simulink model "CTC_3PPP"  (R2018b)
settings: Solver=ode3  StartTime=0.0  StopTime=7  FixedStep=1e-3  RelTol=1e-3  EnableMultiTasking=on
undefined symbols (not defined in the file or in its folder): X, Y, Z
libraries: sm_lib x53, nesl_utility x13, simulink x2
(part 2 of 2)

== system CTC_3PPP/Mechanical/Mechanical/L2_6_RIGID ==
  ReferenceFrame : sm_lib/Frames and Transforms/Reference Frame
  Solid : sm_lib/Body Elements/Solid  InertiaType=Custom  Mass=7.3903600000000003  MassUnits=kg  CenterOfMass=[-300 -10 0]  CenterOfMassUnits=mm  MomentsOfInertia=[4161.6100000000006 267638 263969]  MomentsOfInertiaUnits=kg*mm^2  ProductsOfInertia=[0 0 0]  ProductsOfInertiaUnits=kg*mm^2  BasedOnType=Density  Density=1000  DensityUnits=kg/(m^3)  DoExposeReferenceFrame=on  SerializedFrames=<Frames/>  GraphicType=FromGeometry  MarkerShape=Sphere  MarkerSize=10  MarkerSizeUnits=m  GraphicVisPropType=SimpleVisualProperties  GraphicDiffuseColor=[0.909804 0.443137 0.0313725]  GraphicSpecularColor=[0.5 0.5 0.5 1.0]  GraphicAmbientColor=[0.15 0.15 0.15 1.0]  GraphicEmissiveColor=[0.0 0.0 0.0 1.0]  GraphicShininess=75  GraphicOpacity=1  GeometryShape=FromFile  RectangleSize=[1 1]  RectangleSizeUnits=m  BrickDimensions=[1 1 1]  BrickDimensionUnits=m  CylinderRadius=1  CylinderRadiusUnits=m  CylinderLength=1  CylinderLengthUnits=m  SphereRadius=1  SphereRadiusUnits=m  EllipsoidRadii=[1 1 1]  EllipsoidRadiiUnits=m  ExtrusionCrossSection=[1 1; -1 1; -1 -1; 1 -1]  ExtrusionCrossSectionUnits=m  ExtrusionLength=1  ExtrusionLengthUnits=m  PolygonNumSides=3  PolygonOuterRadius=1  PolygonOuterRadiusUnits=m  ExtGeomFileType=STL  ExtGeomFileName=L2_Default_sldprt.STL  ExtGeomFileUnits=mm  RevolutionCrossSection=[1 1; 1 -1; 2 -1; 2 1]  RevolutionCrossSectionUnits=m  RevolutionExtent=Full  RevolutionAngle=180  RevolutionAngleUnits=deg
  Transform : sm_lib/Frames and Transforms/Rigid Transform  TranslationMethod=Cartesian  TranslationStandardOffset=0  TranslationLengthUnit=mm  TranslationStandardAxis=+Z  TranslationCartesianOffset=[-600.00300519535062 20.000000000004142 -0.0012441245004310986]  TranslationROffset=0  TranslationROffsetUnits=m  TranslationZOffset=0  TranslationZOffsetUnits=m  TranslationThetaOffset=0  TranslationThetaOffsetUnits=deg  RotationMethod=ArbitraryAxis  RotationAngleUnits=rad  RotationStandardAxis=+Z  RotationAngle=2.0943951023931953  RotationArbitraryAxis=[0.57735026918962584 -0.57735026918962595 0.57735026918962573]  FollAlignAxisA=+X  BaseAlignAxisA=+Y  FollAlignAxisB=+Y  BaseAlignAxisB=+Z  RotationSequenceAxes=FollowerAxes  RotationSequence=XYX  RotationSequenceAngles=[0 0 0]  RotationSequenceAnglesUnits=deg  RotationMatrix=[1 0 0; 0 1 0; 0 0 1]
  Transform1 : sm_lib/Frames and Transforms/Rigid Transform  TranslationMethod=Cartesian  TranslationStandardOffset=0  TranslationLengthUnit=mm  TranslationStandardAxis=+Z  TranslationCartesianOffset=[0 0 0]  TranslationROffset=0  TranslationROffsetUnits=m  TranslationZOffset=0  TranslationZOffsetUnits=m  TranslationThetaOffset=0  TranslationThetaOffsetUnits=deg  RotationMethod=ArbitraryAxis  RotationAngleUnits=rad  RotationStandardAxis=+Z  RotationAngle=2.0943951023931953  RotationArbitraryAxis=[0.57735026918962584 -0.57735026918962584 0.57735026918962584]  FollAlignAxisA=+X  BaseAlignAxisA=+Y  FollAlignAxisB=+Y  BaseAlignAxisB=+Z  RotationSequenceAxes=FollowerAxes  RotationSequence=XYX  RotationSequenceAngles=[0 0 0]  RotationSequenceAnglesUnits=deg  RotationMatrix=[1 0 0; 0 1 0; 0 0 1]
  F : PMIOPort  Side=Left
  F1 : PMIOPort  Port=2  Side=Right
  connections:
  Solid/RConn1 -- ReferenceFrame/RConn1 -- Transform/LConn1 -- Transform1/LConn1
  Transform/RConn1 -- F/RConn1
  Transform1/RConn1 -- F1/RConn1

== system CTC_3PPP/Mechanical/Mechanical/de2_5_RIGID ==
  ReferenceFrame : sm_lib/Frames and Transforms/Reference Frame
  Solid : sm_lib/Body Elements/Solid  InertiaType=Custom  Mass=5.2339599999999997  MassUnits=kg  CenterOfMass=[0 145.71899999999999 1.0172299999999999e-12]  CenterOfMassUnits=mm  MomentsOfInertia=[33998.800000000003 21791.899999999998 33998.800000000003]  MomentsOfInertiaUnits=kg*mm^2  ProductsOfInertia=[0 0 0]  ProductsOfInertiaUnits=kg*mm^2  BasedOnType=Density  Density=1000  DensityUnits=kg/(m^3)  DoExposeReferenceFrame=on  SerializedFrames=<Frames/>  GraphicType=FromGeometry  MarkerShape=Sphere  MarkerSize=10  MarkerSizeUnits=m  GraphicVisPropType=SimpleVisualProperties  GraphicDiffuseColor=[0.792157 0.819608 0.933333]  GraphicSpecularColor=[0.5 0.5 0.5 1.0]  GraphicAmbientColor=[0.15 0.15 0.15 1.0]  GraphicEmissiveColor=[0.0 0.0 0.0 1.0]  GraphicShininess=75  GraphicOpacity=1  GeometryShape=FromFile  RectangleSize=[1 1]  RectangleSizeUnits=m  BrickDimensions=[1 1 1]  BrickDimensionUnits=m  CylinderRadius=1  CylinderRadiusUnits=m  CylinderLength=1  CylinderLengthUnits=m  SphereRadius=1  SphereRadiusUnits=m  EllipsoidRadii=[1 1 1]  EllipsoidRadiiUnits=m  ExtrusionCrossSection=[1 1; -1 1; -1 -1; 1 -1]  ExtrusionCrossSectionUnits=m  ExtrusionLength=1  ExtrusionLengthUnits=m  PolygonNumSides=3  PolygonOuterRadius=1  PolygonOuterRadiusUnits=m  ExtGeomFileType=STL  ExtGeomFileName=de2_Default_sldprt.STL  ExtGeomFileUnits=mm  RevolutionCrossSection=[1 1; 1 -1; 2 -1; 2 1]  RevolutionCrossSectionUnits=m  RevolutionExtent=Full  RevolutionAngle=180  RevolutionAngleUnits=deg
  Transform : sm_lib/Frames and Transforms/Rigid Transform  TranslationMethod=Cartesian  TranslationStandardOffset=0  TranslationLengthUnit=mm  TranslationStandardAxis=+Z  TranslationCartesianOffset=[0 0 0]  TranslationROffset=0  TranslationROffsetUnits=m  TranslationZOffset=0  TranslationZOffsetUnits=m  TranslationThetaOffset=0  TranslationThetaOffsetUnits=deg  RotationMethod=ArbitraryAxis  RotationAngleUnits=rad  RotationStandardAxis=+Z  RotationAngle=2.0943951023931913  RotationArbitraryAxis=[-0.57735026918962451 -0.57735026918962451 -0.57735026918962828]  FollAlignAxisA=+X  BaseAlignAxisA=+Y  FollAlignAxisB=+Y  BaseAlignAxisB=+Z  RotationSequenceAxes=FollowerAxes  RotationSequence=XYX  RotationSequenceAngles=[0 0 0]  RotationSequenceAnglesUnits=deg  RotationMatrix=[1 0 0; 0 1 0; 0 0 1]
  F1 : PMIOPort  Side=Left
  F : PMIOPort  Port=2  Side=Right
  connections:
  Solid/RConn1 -- ReferenceFrame/RConn1 -- Transform/LConn1 -- F1/RConn1
  Transform/RConn1 -- F/RConn1

== system CTC_3PPP/Mechanical/Mechanical/de2_6_RIGID ==
  ReferenceFrame : sm_lib/Frames and Transforms/Reference Frame
  Solid : sm_lib/Body Elements/Solid  InertiaType=Custom  Mass=5.2339599999999997  MassUnits=kg  CenterOfMass=[0 145.71899999999999 1.0172299999999999e-12]  CenterOfMassUnits=mm  MomentsOfInertia=[33998.800000000003 21791.899999999998 33998.800000000003]  MomentsOfInertiaUnits=kg*mm^2  ProductsOfInertia=[0 0 0]  ProductsOfInertiaUnits=kg*mm^2  BasedOnType=Density  Density=1000  DensityUnits=kg/(m^3)  DoExposeReferenceFrame=on  SerializedFrames=<Frames/>  GraphicType=FromGeometry  MarkerShape=Sphere  MarkerSize=10  MarkerSizeUnits=m  GraphicVisPropType=SimpleVisualProperties  GraphicDiffuseColor=[0.792157 0.819608 0.933333]  GraphicSpecularColor=[0.5 0.5 0.5 1.0]  GraphicAmbientColor=[0.15 0.15 0.15 1.0]  GraphicEmissiveColor=[0.0 0.0 0.0 1.0]  GraphicShininess=75  GraphicOpacity=1  GeometryShape=FromFile  RectangleSize=[1 1]  RectangleSizeUnits=m  BrickDimensions=[1 1 1]  BrickDimensionUnits=m  CylinderRadius=1  CylinderRadiusUnits=m  CylinderLength=1  CylinderLengthUnits=m  SphereRadius=1  SphereRadiusUnits=m  EllipsoidRadii=[1 1 1]  EllipsoidRadiiUnits=m  ExtrusionCrossSection=[1 1; -1 1; -1 -1; 1 -1]  ExtrusionCrossSectionUnits=m  ExtrusionLength=1  ExtrusionLengthUnits=m  PolygonNumSides=3  PolygonOuterRadius=1  PolygonOuterRadiusUnits=m  ExtGeomFileType=STL  ExtGeomFileName=de2_Default_sldprt.STL  ExtGeomFileUnits=mm  RevolutionCrossSection=[1 1; 1 -1; 2 -1; 2 1]  RevolutionCrossSectionUnits=m  RevolutionExtent=Full  RevolutionAngle=180  RevolutionAngleUnits=deg
  Transform : sm_lib/Frames and Transforms/Rigid Transform  TranslationMethod=Cartesian  TranslationStandardOffset=0  TranslationLengthUnit=mm  TranslationStandardAxis=+Z  TranslationCartesianOffset=[0 0 0]  TranslationROffset=0  TranslationROffsetUnits=m  TranslationZOffset=0  TranslationZOffsetUnits=m  TranslationThetaOffset=0  TranslationThetaOffsetUnits=deg  RotationMethod=ArbitraryAxis  RotationAngleUnits=rad  RotationStandardAxis=+Z  RotationAngle=2.0943951023931913  RotationArbitraryAxis=[-0.57735026918962451 -0.57735026918962451 -0.57735026918962828]  FollAlignAxisA=+X  BaseAlignAxisA=+Y  FollAlignAxisB=+Y  BaseAlignAxisB=+Z  RotationSequenceAxes=FollowerAxes  RotationSequence=XYX  RotationSequenceAngles=[0 0 0]  RotationSequenceAnglesUnits=deg  RotationMatrix=[1 0 0; 0 1 0; 0 0 1]
  F1 : PMIOPort  Side=Left
  F : PMIOPort  Port=2  Side=Right
  connections:
  Solid/RConn1 -- ReferenceFrame/RConn1 -- Transform/LConn1 -- F1/RConn1
  Transform/RConn1 -- F/RConn1

== system CTC_3PPP/Mechanical/Mechanical/de2_7_RIGID ==
  ReferenceFrame : sm_lib/Frames and Transforms/Reference Frame
  Solid : sm_lib/Body Elements/Solid  InertiaType=Custom  Mass=5.2339599999999997  MassUnits=kg  CenterOfMass=[0 145.71899999999999 1.0172299999999999e-12]  CenterOfMassUnits=mm  MomentsOfInertia=[33998.800000000003 21791.899999999998 33998.800000000003]  MomentsOfInertiaUnits=kg*mm^2  ProductsOfInertia=[0 0 0]  ProductsOfInertiaUnits=kg*mm^2  BasedOnType=Density  Density=1000  DensityUnits=kg/(m^3)  DoExposeReferenceFrame=on  SerializedFrames=<Frames/>  GraphicType=FromGeometry  MarkerShape=Sphere  MarkerSize=10  MarkerSizeUnits=m  GraphicVisPropType=SimpleVisualProperties  GraphicDiffuseColor=[0.792157 0.819608 0.933333]  GraphicSpecularColor=[0.5 0.5 0.5 1.0]  GraphicAmbientColor=[0.15 0.15 0.15 1.0]  GraphicEmissiveColor=[0.0 0.0 0.0 1.0]  GraphicShininess=75  GraphicOpacity=1  GeometryShape=FromFile  RectangleSize=[1 1]  RectangleSizeUnits=m  BrickDimensions=[1 1 1]  BrickDimensionUnits=m  CylinderRadius=1  CylinderRadiusUnits=m  CylinderLength=1  CylinderLengthUnits=m  SphereRadius=1  SphereRadiusUnits=m  EllipsoidRadii=[1 1 1]  EllipsoidRadiiUnits=m  ExtrusionCrossSection=[1 1; -1 1; -1 -1; 1 -1]  ExtrusionCrossSectionUnits=m  ExtrusionLength=1  ExtrusionLengthUnits=m  PolygonNumSides=3  PolygonOuterRadius=1  PolygonOuterRadiusUnits=m  ExtGeomFileType=STL  ExtGeomFileName=de2_Default_sldprt.STL  ExtGeomFileUnits=mm  RevolutionCrossSection=[1 1; 1 -1; 2 -1; 2 1]  RevolutionCrossSectionUnits=m  RevolutionExtent=Full  RevolutionAngle=180  RevolutionAngleUnits=deg
  Transform : sm_lib/Frames and Transforms/Rigid Transform  TranslationMethod=Cartesian  TranslationStandardOffset=0  TranslationLengthUnit=mm  TranslationStandardAxis=+Z  TranslationCartesianOffset=[0 0 0]  TranslationROffset=0  TranslationROffsetUnits=m  TranslationZOffset=0  TranslationZOffsetUnits=m  TranslationThetaOffset=0  TranslationThetaOffsetUnits=deg  RotationMethod=ArbitraryAxis  RotationAngleUnits=rad  RotationStandardAxis=+Z  RotationAngle=2.0943951023931913  RotationArbitraryAxis=[-0.57735026918962451 -0.57735026918962451 -0.57735026918962828]  FollAlignAxisA=+X  BaseAlignAxisA=+Y  FollAlignAxisB=+Y  BaseAlignAxisB=+Z  RotationSequenceAxes=FollowerAxes  RotationSequence=XYX  RotationSequenceAngles=[0 0 0]  RotationSequenceAnglesUnits=deg  RotationMatrix=[1 0 0; 0 1 0; 0 0 1]
  F1 : PMIOPort  Side=Left
  F : PMIOPort  Port=2  Side=Right
  connections:
  Solid/RConn1 -- ReferenceFrame/RConn1 -- Transform/LConn1 -- F1/RConn1
  Transform/RConn1 -- F/RConn1

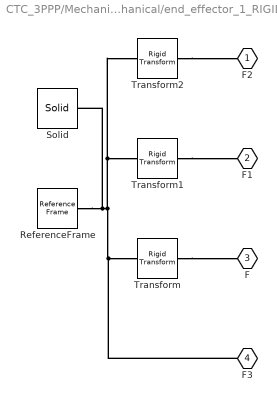
== system CTC_3PPP/Mechanical/Mechanical/end_effector_1_RIGID ==
  ReferenceFrame : sm_lib/Frames and Transforms/Reference Frame
  Solid : sm_lib/Body Elements/Solid  InertiaType=Custom  Mass=3.8378800000000002  MassUnits=kg  CenterOfMass=[0 -7.5 -1.46335e-12]  CenterOfMassUnits=mm  MomentsOfInertia=[32683.700000000004 65223.500000000007 32683.700000000004]  MomentsOfInertiaUnits=kg*mm^2  ProductsOfInertia=[0 0 0]  ProductsOfInertiaUnits=kg*mm^2  BasedOnType=Density  Density=1000  DensityUnits=kg/(m^3)  DoExposeReferenceFrame=on  SerializedFrames=<Frames/>  GraphicType=FromGeometry  MarkerShape=Sphere  MarkerSize=10  MarkerSizeUnits=m  GraphicVisPropType=SimpleVisualProperties  GraphicDiffuseColor=[0.894118 0.913725 0.929412]  GraphicSpecularColor=[0.5 0.5 0.5 1.0]  GraphicAmbientColor=[0.15 0.15 0.15 1.0]  GraphicEmissiveColor=[0.0 0.0 0.0 1.0]  GraphicShininess=75  GraphicOpacity=1  GeometryShape=FromFile  RectangleSize=[1 1]  RectangleSizeUnits=m  BrickDimensions=[1 1 1]  BrickDimensionUnits=m  CylinderRadius=1  CylinderRadiusUnits=m  CylinderLength=1  CylinderLengthUnits=m  SphereRadius=1  SphereRadiusUnits=m  EllipsoidRadii=[1 1 1]  EllipsoidRadiiUnits=m  ExtrusionCrossSection=[1 1; -1 1; -1 -1; 1 -1]  ExtrusionCrossSectionUnits=m  ExtrusionLength=1  ExtrusionLengthUnits=m  PolygonNumSides=3  PolygonOuterRadius=1  PolygonOuterRadiusUnits=m  ExtGeomFileType=STL  ExtGeomFileName=end-effector_Default_sldprt.STL  ExtGeomFileUnits=mm  RevolutionCrossSection=[1 1; 1 -1; 2 -1; 2 1]  RevolutionCrossSectionUnits=m  RevolutionExtent=Full  RevolutionAngle=180  RevolutionAngleUnits=deg
  Transform : sm_lib/Frames and Transforms/Rigid Transform  TranslationMethod=Cartesian  TranslationStandardOffset=0  TranslationLengthUnit=mm  TranslationStandardAxis=+Z  TranslationCartesianOffset=[-173.2045872608081 -15.00000000000081 -99.999473127677447]  TranslationROffset=0  TranslationROffsetUnits=m  TranslationZOffset=0  TranslationZOffsetUnits=m  TranslationThetaOffset=0  TranslationThetaOffsetUnits=deg  RotationMethod=ArbitraryAxis  RotationAngleUnits=rad  RotationStandardAxis=+Z  RotationAngle=2.0943951023931953  RotationArbitraryAxis=[0.57735026918962584 -0.57735026918962584 0.57735026918962584]  FollAlignAxisA=+X  BaseAlignAxisA=+Y  FollAlignAxisB=+Y  BaseAlignAxisB=+Z  RotationSequenceAxes=FollowerAxes  RotationSequence=XYX  RotationSequenceAngles=[0 0 0]  RotationSequenceAnglesUnits=deg  RotationMatrix=[1 0 0; 0 1 0; 0 0 1]
  Transform1 : sm_lib/Frames and Transforms/Rigid Transform  TranslationMethod=Cartesian  TranslationStandardOffset=0  TranslationLengthUnit=mm  TranslationStandardAxis=+Z  TranslationCartesianOffset=[173.20555958822573 -15.000000000000609 -99.999297526180612]  TranslationROffset=0  TranslationROffsetUnits=m  TranslationZOffset=0  TranslationZOffsetUnits=m  TranslationThetaOffset=0  TranslationThetaOffsetUnits=deg  RotationMethod=ArbitraryAxis  RotationAngleUnits=rad  RotationStandardAxis=+Z  RotationAngle=2.0943951023931957  RotationArbitraryAxis=[0.57735026918962573 -0.57735026918962573 0.57735026918962584]  FollAlignAxisA=+X  BaseAlignAxisA=+Y  FollAlignAxisB=+Y  BaseAlignAxisB=+Z  RotationSequenceAxes=FollowerAxes  RotationSequence=XYX  RotationSequenceAngles=[0 0 0]  RotationSequenceAnglesUnits=deg  RotationMatrix=[1 0 0; 0 1 0; 0 0 1]
  Transform2 : sm_lib/Frames and Transforms/Rigid Transform  TranslationMethod=Cartesian  TranslationStandardOffset=0  TranslationLengthUnit=mm  TranslationStandardAxis=+Z  TranslationCartesianOffset=[0.00019460048216402015 -14.999999999998581 200.00067808125598]  TranslationROffset=0  TranslationROffsetUnits=m  TranslationZOffset=0  TranslationZOffsetUnits=m  TranslationThetaOffset=0  TranslationThetaOffsetUnits=deg  RotationMethod=ArbitraryAxis  RotationAngleUnits=rad  RotationStandardAxis=+Z  RotationAngle=2.0943951023931953  RotationArbitraryAxis=[0.57735026918962584 -0.57735026918962584 0.57735026918962584]  FollAlignAxisA=+X  BaseAlignAxisA=+Y  FollAlignAxisB=+Y  BaseAlignAxisB=+Z  RotationSequenceAxes=FollowerAxes  RotationSequence=XYX  RotationSequenceAngles=[0 0 0]  RotationSequenceAnglesUnits=deg  RotationMatrix=[1 0 0; 0 1 0; 0 0 1]
  F2 : PMIOPort  Side=Left
  F1 : PMIOPort  Port=2  Side=Left
  F : PMIOPort  Port=3  Side=Left
  F3 : PMIOPort  Port=4  Side=Right
  connections:
  Solid/RConn1 -- ReferenceFrame/RConn1 -- Transform1/LConn1 -- Transform2/LConn1 -- F3/RConn1 -- Transform/LConn1
  Transform/RConn1 -- F/RConn1
  Transform1/RConn1 -- F1/RConn1
  Transform2/RConn1 -- F2/RConn1

== matlab function CTC_3PPP/MATLAB Function1 ==
  data: x output; teta1 input; y output; teta2 input; teta3 input; goc output; phi1 output; phi2 output; phi3 output
function  [x,y,goc,phi1,phi2,phi3]=forward1(teta1,teta2,teta3)
%% Thong so
l1=0.4;
l2=0.6;
l3=0.2;
%%
phii=[pi/6 5*pi/6 3*pi/2];
xoi=[0 1 0.5];
yoi=[0 0 sqrt(3)/2];

gama1=7*pi/6;
gama2=11*pi/6;
gama3=pi/2;
gama=[gama1; gama2; gama3;];
%%
z2=[0;0;0;];

%% giai phuong trinh tai day
coder.extrinsic('giaihe') %% chuyen C++ => matlab function
z2=giaihe(teta1,teta2,teta3);
x=z2(1);
y=z2(2);
goc=z2(3);
tam=[0; 0; 0;];
%% Tinh phi
phi=[0; 0; 0;];
xci=[0; 0; 0;];
yci=[0; 0; 0;];
for i=1:3
    xci(i)=x+l3*cos(goc+gama(i))-xoi(i);
    yci(i)=y+l3*sin(goc+gama(i))-yoi(i);
    tam(i)=(l1^2+l2^2-xci(i)^2-yci(i)^2)/(2*l1*l2);
    phi(i)=acos(tam(i))-pi;
end
%%
xc1=xci(1);
xc2=xci(2);
xc3=xci(3);
yc1=yci(1);
yc2=yci(2);
yc3=yci(3);
phi1=phi(1);
phi2=phi(2);
phi3=phi(3);

== matlab function CTC_3PPP/Mechanical/Mechanical/Coulomb & Viscous Friction3/Embedded MATLAB Function ==
  data: u input; y output
function y = Sat(u)

if (abs(u)>0.01)
    y = sign(u);
else
    y = u/0.01;
end

== matlab function CTC_3PPP/Mechanical/Mechanical/Coulomb & Viscous Friction1/Embedded MATLAB Function ==
  data: u input; y output
function y = Sat(u)

if (abs(u)>0.01)
    y = sign(u);
else
    y = u/0.01;
end

== matlab function CTC_3PPP/Mechanical/Mechanical/Coulomb & Viscous Friction2/Embedded MATLAB Function ==
  data: u input; y output
function y = Sat(u)

if (abs(u)>0.01)
    y = sign(u);
else
    y = u/0.01;
end

== matlab function CTC_3PPP/MATLAB Function2 ==
  settings: updateMethod=DISCRETE
  data: xp input; To1 output; yp input; anpha input; teta1 input; teta2 input; teta3 input; phi1 input; phi2 input; phi3 input; teta1_dot input; teta2_dot input; teta3_dot input; teta1d input; teta2d input; teta3d input; teta1d_dot input; teta2d_dot input; teta3d_dot input; teta1d_2dot input; teta2d_2dot input; teta3d_2dot input; To2 output; To3 output
function [To1,To2,To3] = Dynamic(xp,yp,anpha,teta1,teta2,teta3,phi1,phi2,phi3,teta1_dot,teta2_dot,teta3_dot,teta1d,teta2d,teta3d,teta1d_dot,teta2d_dot,teta3d_dot,teta1d_2dot,teta2d_2dot,teta3d_2dot)


%% Thong so
l1=0.4;
l2=0.6;
l3=0.2;
%%
gama1=pi/6+anpha;
gama2=5*pi/6+anpha;
gama3=3*pi/2+anpha;
gama=[gama1; gama2; gama3;];

%%
m1=5.11836;I1=91391*10^-6;% kg/m^2;
m2=7.39036;I2=267638*10^-6; % kg/m^2;
mp=3.83788; Ip=65223*10^-6% % kg/m^2; - end-effector

%%
xoi=[0 1 0.5];
yoi=[0 0 sqrt(3)/2];
%%
tetaout1=teta1;
tetaout2=teta2;
tetaout3=teta3;
%%
teta=[teta1; teta2; teta3;];
phi=[phi1; phi2; phi3;];
z=[xp; yp; anpha;];
z_dot=[0; 0; 0;];
z_2dot=[0; 0; 0;];
%%
teta_dot=[teta1_dot; teta2_dot; teta3_dot;];
teta_2dot=[0; 0; 0;];
%% Tinh Jz1*z_dot=Jo*teta_dot;
%% z_dot= inv(Jz1)*Jo*teta_dot
az1=[0 0 0];
bz1=[0 0 0];
cz1=[0 0 0];
dz1=[0 0 0];

for i=1:3
    az1(i)=cos(teta(i)+phi(i));
    bz1(i)=sin(teta(i)+phi(i));
    cz1(i)=-l3*sin(teta(i)+phi(i)-gama(i));
    dz1(i)=l1*sin(phi(i));
end
Jz1=[az1(1) bz1(1) cz1(1);
     az1(2) bz1(2) cz1(2);
     az1(3) bz1(3) cz1(3);];
 Jo=[dz1(1) 0 0;
     0 dz1(2) 0;
     0 0 dz1(3);];
 
z_dot=inv(Jz1)*Jo*teta_dot;
xp_dot=z_dot(1);
yp_dot=z_dot(2);
anpha_dot=z_dot(3);
 %% Tinh Jz2*z_dot=Jp*phi_dot
az2=[0 0 0];
bz2=[0 0 0];
cz2=[0 0 0];
dz2=[0 0 0];
phi_dot=[0; 0; 0;];
for i=1:3
    az2(i)=l1*cos(teta(i))+l2*cos(teta(i)+phi(i));
    bz2(i)=l1*sin(teta(i))+l2*sin(teta(i)+phi(i));
    cz2(i)=l1*l3*sin(gama(i)-teta(i))+l2*l3*sin(gama(i)-teta(i)-phi(i));
    dz2(i)=-l1*l2*sin(phi(i));
end
Jz2=[az2(1) bz2(1) cz2(1);
     az2(2) bz2(2) cz2(2);
     az2(3) bz2(3) cz2(3);];
 Jp=[dz2(1) 0 0;
     0 dz2(2) 0;
     0 0 dz2(3);];
 phi_dot=inv(Jp)*Jz2*z_dot;
 
 %% Jz1_dot, Jz2_dot, Jo_dot, Jp_dot
 az1_dot=[0 0 0];
 bz1_dot=[0 0 0];
 cz1_dot=[0 0 0];
 dz1_dot=[0 0 0];
  for i=1:3
     az1_dot(i)=-sin(teta(i)+phi(i))*(teta_dot(i)+phi_dot(i));
     bz1_dot(i)=cos(teta(i)+phi(i))*(teta_dot(i)+phi_dot(i));
     cz1_dot(i)=-l3*cos(teta(i)+phi(i)-gama(i))*(teta_dot(i)+phi_dot(i)-anpha_dot);
     dz1_dot(i)=l1*cos(phi(i))*phi_dot(i);
 end
 Jz1_dot=[az1_dot(1) bz1_dot(1) cz1_dot(1);
          az1_dot(2) bz1_dot(2) cz1_dot(2);
          az1_dot(3) bz1_dot(3) cz1_dot(3);];
 Jo_dot=[dz1_dot(1) 0 0;
         0 dz1_dot(2) 0;
         0 0 dz1_dot(3);];
 az2_dot=[0 0 0];
 bz2_dot=[0 0 0];
 cz2_dot=[0 0 0];
 dz2_dot=[0 0 0];
 for i=1:3
     az2_dot(i)=-l1*sin(teta(i))*teta_dot(i)-l2*sin(teta(i)+phi(i))*(teta_dot(i)+phi_dot(i));
     bz2_dot(i)=l1*cos(teta(i))*teta_dot(i)+l2*cos(teta(i)+phi(i))*(teta_dot(i)+phi_dot(i));
     cz2_dot(i)=l1*l3*cos(gama(i)-teta(i))*(anpha_dot-teta_dot(i))+l2*l3*cos(gama(i)-teta(i)-phi(i))*(anpha_dot-teta_dot(i)-phi_dot(i));
     dz2_dot(i)=-l1*l2*cos(phi(i))*phi_dot(i);
 end
 Jz2_dot=[az2_dot(1) bz2_dot(1) cz2_dot(1);
          az2_dot(2) bz2_dot(2) cz2_dot(2);
          az2_dot(3) bz2_dot(3) cz2_dot(3);];
 Jp_dot=[dz2_dot(1) 0 0;
         0 dz2_dot(2) 0;
         0 0 dz2_dot(3);];
 %teta_2dot=inv(Jo)*(Jz1_dot*z_dot+Jz1*z_2dot-Jo_dot*teta_dot);

%% Dynamic
lc1=l1/2;
lc2=l2/2;
anphai=m1*lc1^2+m2*l1^2+I1;
betai=m2*lc2^2+I2;
gamai=m2*l1*lc2;

  c2i=cos(phi);
  s2i=sin(phi);
 

Mq=[anphai+betai+2*gamai*c2i(1)              0                      0                  betai+gamai*c2i(1)          0              0             0 0 0;
            0                 anphai+betai+2*gamai*c2i(2)           0                           0        betai+gamai*c2i(2)       0             0 0 0;
            0                               0            anphai+betai+2*gamai*c2i(2)            0                   0      betai+gamai*c2i(3)   0 0 0;
     betai+gamai*c2i(1)                     0                       0                           betai               0              0            0 0 0;
            0                      betai+gamai*c2i(2)               0                           0                   betai          0            0 0 0;
            0                               0               betai+gamai*c2i(3)                  0                   0            betai          0 0 0;
            0                               0                       0                           0                   0               0           mp 0 0;
            0                               0                       0                           0                   0               0           0 mp 0;
            0                               0                       0                           0                   0               0           0 0 Ip;];
   
   
Cq=[-2*gamai*phi_dot(1)*s2i(1)          0             0           -gamai*phi_dot(1)*s2i(1)              0                0               0 0 0;
              0          -2*gamai*phi_dot(2)*s2i(2)   0                     0              -gamai*phi_dot(2)*s2i(2)      0               0 0 0;
              0                    0       -2*gamai*phi_dot(3)*s2i(3)       0                       0        -gamai*phi_dot(3)*s2i(3)    0 0 0;
        gamai*teta_dot(1)*s2i(1)   0                  0                     0                       0                    0               0 0 0;
              0       gamai*teta_dot(2)*s2i(2)        0                     0                       0                    0               0 0 0;
              0                    0       gamai*teta_dot(3)*s2i(3)         0                       0                    0               0 0 0;
              0 0 0 0 0 0 0 0 0;
              0 0 0 0 0 0 0 0 0;
              0 0 0 0 0 0 0 0 0;];
 %% Jc_dot=(Jap_dot*Jx-Jp*Jx_dot)/Jx^2

  %% Dynamic
% teta_dot/z_dot=Jz1*inv(Jo)=Joz
% phi_dot/z_dot=Jz2*inv(Jp)=Jpz
Joz=inv(Jo)*Jz1;
Jpz=inv(Jp)*Jz2;
Joz_dot=inv(Jo^2)*(Jz1_dot*Jo-Jz1*Jo_dot);
Jpz_dot=inv(Jp^2)*(Jz2_dot*Jp-Jz1*Jp_dot);

J1=inv(Joz)*Jpz;
J2=inv(Joz);
J1_dot=inv(Joz^2)*(Jpz_dot*Joz-Jpz*Joz_dot);
J2_dot=inv(Joz^2)*Joz_dot;
I=[1 0 0;
   0 1 0;
   0 0 1;];
I_dot=[0 0 0;
       0 0 0;
       0 0 0;];
W=[I;
   J1;
   J2;];

W_dot=[I_dot;
       J1_dot;
       J2_dot;];
M=W'*Mq*W;
C=W'*Mq*W_dot+W'*Cq*W;
%% ------------------------------------------------------------------------
%%  Computed torque control
tetad=[teta1d;
       teta2d;
       teta3d;];
tetad_dot=[teta1d_dot;
           teta2d_dot;
           teta3d_dot;];
tetad_2dot=[teta1d_2dot;
           teta2d_2dot;
           teta3d_2dot;];
 tetar_dot=[0; 0; 0;];
 tetar_2dot=[0; 0; 0;];
 To_a=[0; 0; 0;];
% Position Error
et=[0; 0; 0;];
for i=1:3,
    et(i)=tetad(i)-teta(i);
end 
% Velocity error
et_dot=[0; 0; 0;];
for i=1:3,
    et_dot(i)=tetad_dot(i)-teta_dot(i);
end 
%--------------CTC------------
K1=[25 0 0;
    0 25 0;
    0 0 25;];

K2=[50 0 0;
    0 50 0;
    0 0 50;];

%--------------------------------------------------------------------------
%--------------------------------------------------------------------------
To_a=M*(tetad_2dot+K1*et_dot+K2*et)+C*teta_dot;
To1=To_a(1);
To2=To_a(2);
To3=To_a(3);

== matlab function CTC_3PPP/Inverse3/Invers ==
  data: x input; y input; anpha input; teta1 output; teta2 output; teta3 output; passi1 output; passi2 output; passi3 output; xc1 output; yc1 output; xc2 output; yc2 output; xc3 output; yc3 output
function [teta1,teta2,teta3,passi1,passi2,passi3,xc1,yc1,xc2,yc2,xc3,yc3]   =newkinematic(x,y,anpha)
%% Thong so
l1=0.4;
l2=0.6;
l3=0.2;
%%
phi1=7*pi/6+anpha;
phi2=11*pi/6+anpha;
phi3=pi/2+anpha;
phi=[phi1 phi2 phi3];
%%
xoi=[0 1 0.5];
yoi=[0 0 sqrt(3)/2];
%%
si=[0 0 0];
betai=[0 0 0];
xci=[0 0 0];
yci=[0 0 0];
teta=[0 0 0];
passi=[0 0 0];
tam=[0 0 0];
tam1=[0 0 0];
canh2p=[0 0 0];
canh=[0 0 0];

for i=1:3
    xci(i)=x+l3*cos(phi(i))-xoi(i);
    yci(i)=y+l3*sin(phi(i))-yoi(i);
    si(i)=atan2(yci(i),xci(i));
    canh2p(i)=xci(i)^2+yci(i)^2;
    canh(i)=sqrt(canh2p(i));
    tam1(i)=(l1^2-l2^2+canh2p(i))/(2*l1*canh(i));
   
    betai(i)=acos(tam1(i));
    teta(i)=si(i)+betai(i);
    if teta(i)>2*pi
        teta(i)=teta(i)-2*pi;
    end
    
   passi(i)=acos((l1^2+l2^2-canh2p(i))/(2*l1*l2))-pi;
end


teta1=teta(1);
teta2=teta(2);
teta3=teta(3);
passi1=passi(1);
passi2=passi(2);
passi3=passi(3);
%%
xc1=si(1);
xc2=si(2);
xc3=si(3);

yc1=betai(1);
yc2=betai(2);
yc3=betai(3);

== matlab function CTC_3PPP/Jacobian4/Jacobian1 ==
  data: teta1_out output; teta2_out output; teta3_out output; xp input; teta1_dot output; yp input; anpha input; teta1 input; teta2 input; teta3 input; phi1 input; phi2 input; phi3 input; xp_dot input; yp_dot input; anpha_dot input; xp_2dot input; yp_2dot input; anpha_2dot input; teta2_dot output; teta3_dot output; teta1_2dot output; teta2_2dot output; teta3_2dot output
function [teta1_out,teta2_out,teta3_out,teta1_dot,teta2_dot,teta3_dot,teta1_2dot,teta2_2dot,teta3_2dot] = Jacobian(xp,yp,anpha,teta1,teta2,teta3,phi1,phi2,phi3,xp_dot,yp_dot,anpha_dot,xp_2dot,yp_2dot,anpha_2dot)
%% Thong so
l1=0.4;
l2=0.6;
l3=0.2;

anpha1=anpha+pi/6;
anpha2=anpha+5*pi/6;
anpha3=anpha-pi/2;
anphai=[anpha1 anpha2 anpha3];

xoi=[0 1 0.5];
yoi=[0 0 sqrt(3)/2];

z=[xp yp anpha];
teta=[teta1 teta2 teta3];
phi=[phi1 phi2 phi3];

z_dot=[xp_dot yp_dot anpha_dot];
z_dd=[xp_2dot yp_2dot anpha_2dot];

teta_dot=[0 0 0];
teta_2dot=[0; 0 ;0;];
teta1_out=teta1;
teta2_out=teta2;
teta3_out=teta3;
%%
%% Jz*Z'=Jo*O'
betai=[0 0 0];
for i=1:3
    betai(i)=teta(i)+phi(i);
end
Jz=[cos(betai(1)) sin(betai(1)) -l3*sin(betai(1)-(anphai(1)));
    cos(betai(2)) sin(betai(2)) -l3*sin(betai(2)-(anphai(2)));
    cos(betai(3)) sin(betai(3)) -l3*sin(betai(3)-(anphai(3)));];
Jo=[l1*sin(phi(1)) 0 0;
    0 l1*sin(phi(2)) 0 ;
    0 0 l1*sin(phi(3));];
z_dot=z_dot';
teta_dot=teta_dot';
%teta_dot=inv(Jo)*Jz*z_dot;
%% O'=J*Z'
J=inv(Jo)*Jz;
teta_dot=J*z_dot;
teta1_dot=teta_dot(1);
teta2_dot=teta_dot(2);
teta3_dot=teta_dot(3);
%%
%% Phi'=Jp*Z'
a=[0 0 0];
b=[0 0 0];
c=[0 0 0];
d=[0 0 0];
for i=1:3
    a(i)=l1*cos(teta(i))+l2*cos(teta(i)+phi(i));
    b(i)=l1*sin(teta(i))+l2*sin(teta(i)+phi(i));
    c(i)=l1*l3*sin(teta(i)-anphai(i));
    d(i)=-l1*l2*sin(phi(i));
end
Jp=[a(1)/d(1) b(1)/d(1) c(1)/d(1);
    a(2)/d(2) b(2)/d(2) c(2)/d(2);
    a(3)/d(3) b(3)/d(3) c(3)/d(3);];
phi_dot=[0; 0; 0;];
phi_dot=Jp*z_dot;

%%
%% teta_2dot=J'*Z'+J*Z''
a=[Jz(1,1) Jz(1,2) Jz(1,3)];
b=[Jz(2,1) Jz(2,2) Jz(2,3)];
c=[Jz(3,1) Jz(3,2) Jz(3,3)];
d=[Jo(1,1) Jo(2,2) Jo(3,3)];
a_dot=[0 0 0];
b_dot=[0 0 0];
c_dot=[0 0 0];
d_dot=[0 0 0];
for i=1:3
    a_dot(i)=-sin(betai(i))*(teta_dot(i)+phi_dot(i));
    b_dot(i)=cos(betai(i))*(teta_dot(i)+phi_dot(i));
    c_dot(i)=-l3*cos(betai(i)-(anphai(i)))*(teta_dot(i)+phi_dot(i)-anpha_dot);
    d_dot(i)=l1*cos(phi(i))*phi_dot(i);
end

J_dot=[0 0 0;
       0 0 0;
        0 0 0;];
J_dot(1,1)=(a_dot(1)*d(1)-a(1)*d_dot(1))/d(1)^2;
J_dot(1,2)=(a_dot(2)*d(1)-a(2)*d_dot(1))/d(1)^2;
J_dot(1,3)=(a_dot(3)*d(1)-a(3)*d_dot(1))/d(1)^2;

J_dot(2,1)=(a_dot(1)*d(2)-a(1)*d_dot(2))/d(2)^2;
J_dot(2,2)=(a_dot(2)*d(2)-a(2)*d_dot(2))/d(2)^2;
J_dot(2,3)=(a_dot(3)*d(2)-a(3)*d_dot(2))/d(2)^2;

J_dot(3,1)=(a_dot(1)*d(3)-a(1)*d_dot(3))/d(3)^2;
J_dot(3,2)=(a_dot(2)*d(3)-a(2)*d_dot(3))/d(3)^2;
J_dot(3,3)=(a_dot(3)*d(3)-a(3)*d_dot(3))/d(3)^2;

teta_2dot=J_dot*z_dot+J*z_dd';
teta1_2dot=teta_2dot(1);
teta2_2dot=teta_2dot(2);
teta3_2dot=teta_2dot(3);
